simulink model "trajectory"  (R2017b)
settings: Solver=ode45  StartTime=0.0  StopTime=7  RelTol=1e-3
values from neighbouring files (symbols this model uses):
  L = 1.760    (= 1.76)    [Parameters.m]
libraries: simulink x2
settings Model: Creator=Eugene  LastModifiedBy=Eugene
settings DebuggingCC: ParameterOverflowMsg=warning

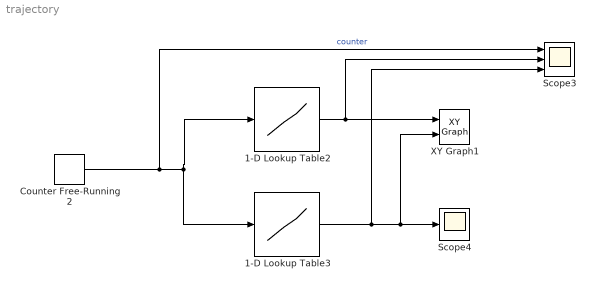
== system trajectory ==
  1-D Lookup Table2 : Lookup_n-D  NumberOfTableDimensions=1  BreakpointsForDimension1=[0:7]  BreakpointsForDimension1FirstPoint=0  BreakpointsForDimension1DataTypeStr=uint8  Table=[0,0,L,L,2*L,2*L,3*L, 3*L]  TableDataTypeStr=double  InterpMethod=Flat  ExtrapMethod=Cubic spline  RemoveProtectionInput=on  InternalRulePriority=Speed  OutDataTypeStr=double  RndMeth=Zero  InputSameDT=on
  1-D Lookup Table3 : Lookup_n-D  NumberOfTableDimensions=1  BreakpointsForDimension1=[0:7]  BreakpointsForDimension1DataTypeStr=int16  Table=[0,25,25,0,0,25,25,0]  TableDataTypeStr=double  InterpMethod=Flat  RemoveProtectionInput=on  InternalRulePriority=Speed  OutDataTypeStr=double  RndMeth=Zero  InputSameDT=on
  Counter Free-Running2 : simulink/Sources/Counter Free-Running  NumBits=3  tsamp=1
  Scope3 : Scope  NumInputPorts=3
  Scope4 : Scope
  XY Graph1 : simulink/Sinks/XY Graph  xmin=-10  xmax=20  ymin=-10  ymax=30  st=-1
  wires:
  1-D Lookup Table3/1 -> Scope4/1, XY Graph1/2, Scope3/3
  1-D Lookup Table2/1 -> XY Graph1/1, Scope3/2
  Counter Free-Running2/1 -> Scope3/1, 1-D Lookup Table2/1, 1-D Lookup Table3/1  "counter"
